simulink model "test"  (R2021b)
settings: Solver=VariableStepAuto  StartTime=0.0  StopTime=30  RelTol=1e-3
settings Model: Creator=lenna  LastModifiedBy=lenna

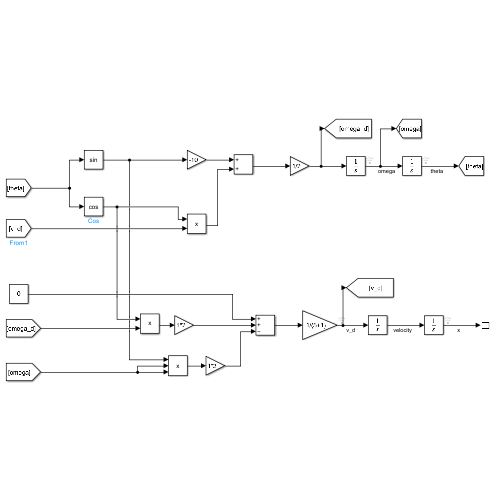
[thumbnail: Simulink's stored preview of the top-level diagram]
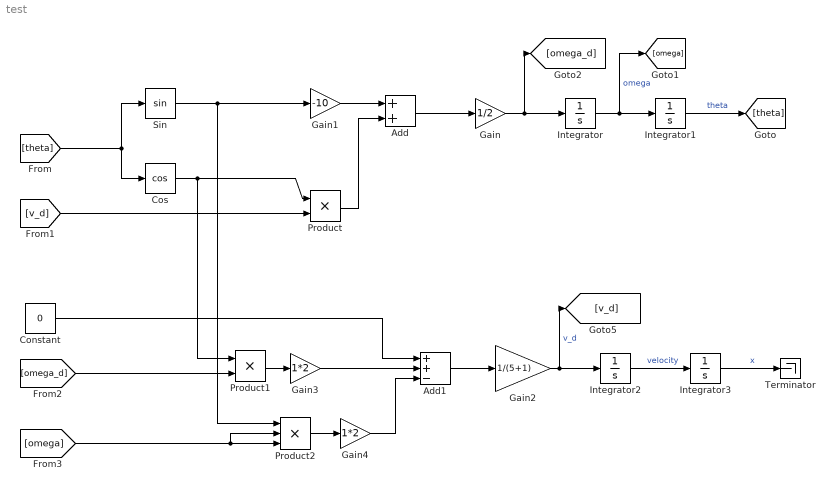
== system test ==
  Add : Sum
  Add1 : Sum  Inputs=++-
  Constant : Constant  Value=0
  Cos : Trigonometry  Operator=cos
  Gain : Gain  Gain=1/2
  Gain1 : Gain  Gain=-10
  Gain2 : Gain  Gain=1/(5+1)
  Gain3 : Gain  Gain=1*2
  Gain4 : Gain  Gain=1*2
  Integrator{,1..3} (4 alike) : Integrator
  Product : Product
  Product1 : Product
  Product2 : Product  Inputs=3
  Sin : Trigonometry
  Terminator : Terminator
  wires:
  Integrator/1 -> [omega], Integrator1/1  "omega"
  Integrator1/1 -> [theta]  "theta"
  Gain/1 -> [omega_d], Integrator/1
  Add/1 -> Gain/1
  [theta] -> Cos/1, Sin/1
  Cos/1 -> Product1/1, Product/1
  [v_d] -> Product/2
  Product/1 -> Add/2
  Gain1/1 -> Add/1
  Constant/1 -> Add1/1
  Add1/1 -> Gain2/1
  Gain2/1 -> [v_d], Integrator2/1  "v_d"
  Product1/1 -> Gain3/1
  Integrator2/1 -> Integrator3/1  "velocity"
  Integrator3/1 -> Terminator/1  "x"
  [omega_d] -> Product1/2
  Gain3/1 -> Add1/2
  Product2/1 -> Gain4/1
  Gain4/1 -> Add1/3
  Sin/1 -> Product2/1, Gain1/1
  [omega] -> Product2/3, Product2/2
